simulink model "MSBR_Plant"  (R2021b)
settings: Solver=ode45  StartTime=0.0  StopTime=sim_time  MaxStep=ts_max  RelTol=1e-4
values from neighbouring files (symbols this model uses):
  a_1 = 8.7292e-2/wilson_ratio    (= 0.0087292)    [Whole_Plant_Cool_Pump_Accident_script.m]    (also in Whole_Plant_Fert_Pump_Accident_script.m; Whole_Plant_Fuel_Pump_Accident.m; Whole_Plant_Fuel_Pump_Accident_script.m; Whole_Plant_Reactivity_Accident.m)
  a_2 = 7.3787e-4/wilson_ratio    (= 7.3787e-05)    [Whole_Plant_Cool_Pump_Accident_script.m]    (also in Whole_Plant_Fert_Pump_Accident_script.m; Whole_Plant_Fuel_Pump_Accident.m; Whole_Plant_Fuel_Pump_Accident_script.m; Whole_Plant_Reactivity_Accident.m)
  a_b = 1.656e-5    (= 1.656e-05)    [Whole_Plant_Cool_Pump_Accident_script.m]    (also in Whole_Plant_Fert_Pump_Accident_script.m; Whole_Plant_Fuel_Pump_Accident.m; Whole_Plant_Fuel_Pump_Accident_script.m; Whole_Plant_Reactivity_Accident.m)
  a_f = -8.172e-5    (= -8.172e-05)    [Whole_Plant_Cool_Pump_Accident_script.m]    (also in Whole_Plant_Fert_Pump_Accident_script.m; Whole_Plant_Fuel_Pump_Accident.m; Whole_Plant_Fuel_Pump_Accident_script.m; Whole_Plant_Reactivity_Accident.m)
  a_g = 2.016e-5    (= 2.016e-05)    [Whole_Plant_Cool_Pump_Accident_script.m]    (also in Whole_Plant_Fert_Pump_Accident_script.m; Whole_Plant_Fuel_Pump_Accident.m; Whole_Plant_Fuel_Pump_Accident_script.m; Whole_Plant_Reactivity_Accident.m)
  A_s = pi()*((D_OTSG_i^2)/4) - A_w_OTSG - A_p_OTSG    [Whole_Plant_Cool_Pump_Accident_script.m]    (also in Whole_Plant_Fert_Pump_Accident_script.m; Whole_Plant_Fuel_Pump_Accident.m; Whole_Plant_Fuel_Pump_Accident_script.m; Whole_Plant_Reactivity_Accident.m)
  alpha_co = 316.2    [Whole_Plant_Cool_Pump_Accident_script.m]    (also in Whole_Plant_Fert_Pump_Accident_script.m; Whole_Plant_Fuel_Pump_Accident.m; Whole_Plant_Fuel_Pump_Accident_script.m; Whole_Plant_Reactivity_Accident.m)
  beta = [2.290e-04, 8.320e-04, 7.100e-04, 8.520e-04, 1.710e-04, 1.020e-04]    [Whole_Plant_Cool_Pump_Accident_script.m]    (also in Whole_Plant_Fert_Pump_Accident_script.m; Whole_Plant_Fuel_Pump_Accident.m; Whole_Plant_Fuel_Pump_Accident_script.m; Whole_Plant_Reactivity_Accident.m)
  beta_co = 68.0958    [Whole_Plant_Cool_Pump_Accident_script.m]    (also in Whole_Plant_Fert_Pump_Accident_script.m; Whole_Plant_Fuel_Pump_Accident.m; Whole_Plant_Fuel_Pump_Accident_script.m; Whole_Plant_Reactivity_Accident.m)
  beta_t = sum(beta)    [Whole_Plant_Cool_Pump_Accident_script.m]    (also in Whole_Plant_Fert_Pump_Accident_script.m; Whole_Plant_Fuel_Pump_Accident.m; Whole_Plant_Fuel_Pump_Accident_script.m; Whole_Plant_Reactivity_Accident.m)
  C_nc_X_A_nc = 12.8    [Whole_Plant_Cool_Pump_Accident_script.m]    (also in Whole_Plant_Fert_Pump_Accident_script.m; Whole_Plant_Fuel_Pump_Accident.m; Whole_Plant_Fuel_Pump_Accident_script.m; Whole_Plant_Reactivity_Accident.m)
  C_pcw = 0.0042    [Whole_Plant_Cool_Pump_Accident_script.m]    (also in Whole_Plant_Fert_Pump_Accident_script.m; Whole_Plant_Fuel_Pump_Accident.m; Whole_Plant_Fuel_Pump_Accident_script.m; Whole_Plant_Reactivity_Accident.m)
  C_rh_X_A_rh = 33    [Whole_Plant_Cool_Pump_Accident_script.m]    (also in Whole_Plant_Fert_Pump_Accident_script.m; Whole_Plant_Fuel_Pump_Accident.m; Whole_Plant_Fuel_Pump_Accident_script.m; Whole_Plant_Reactivity_Accident.m)
  C_v = 0.84    [Whole_Plant_Cool_Pump_Accident_script.m]    (also in Whole_Plant_Fert_Pump_Accident_script.m; Whole_Plant_Fuel_Pump_Accident.m; Whole_Plant_Fuel_Pump_Accident_script.m; Whole_Plant_Reactivity_Accident.m)
  ce1 = 1.2471e-07    [Whole_Plant_Cool_Pump_Accident_script.m]    (also in Whole_Plant_Fert_Pump_Accident_script.m; Whole_Plant_Fuel_Pump_Accident.m; Whole_Plant_Fuel_Pump_Accident_script.m; Whole_Plant_Reactivity_Accident.m)
  ce2 = 5.3816e-14    [Whole_Plant_Cool_Pump_Accident_script.m]    (also in Whole_Plant_Fert_Pump_Accident_script.m; Whole_Plant_Fuel_Pump_Accident.m; Whole_Plant_Fuel_Pump_Accident_script.m; Whole_Plant_Reactivity_Accident.m)
  ce3 = 3.3721e-08    [Whole_Plant_Cool_Pump_Accident_script.m]    (also in Whole_Plant_Fert_Pump_Accident_script.m; Whole_Plant_Fuel_Pump_Accident.m; Whole_Plant_Fuel_Pump_Accident_script.m; Whole_Plant_Reactivity_Accident.m)
  Cp_fw = XSteam('Cp_pT',P_set*10,T_fw)/1000    [Whole_Plant_Cool_Pump_Accident_script.m]    (also in Whole_Plant_Fert_Pump_Accident_script.m; Whole_Plant_Fuel_Pump_Accident.m; Whole_Plant_Fuel_Pump_Accident_script.m; Whole_Plant_Reactivity_Accident.m)
  Cp_p = Cp_sec    (= 0.001716588)    [Whole_Plant_Cool_Pump_Accident_script.m]    (also in Whole_Plant_Fert_Pump_Accident_script.m; Whole_Plant_Fuel_Pump_Accident.m; Whole_Plant_Fuel_Pump_Accident_script.m; Whole_Plant_Reactivity_Accident.m)
  Cp_rh = 0.0021520    (= 0.002152)    [Whole_Plant_Cool_Pump_Accident_script.m]    (also in Whole_Plant_Fert_Pump_Accident_script.m; Whole_Plant_Fuel_Pump_Accident.m; Whole_Plant_Fuel_Pump_Accident_script.m; Whole_Plant_Reactivity_Accident.m)
  Cp_s = XSteam('Cp_pT',P_s*10,T_s)/1000    [Whole_Plant_Cool_Pump_Accident_script.m]    (also in Whole_Plant_Fert_Pump_Accident_script.m; Whole_Plant_Fuel_Pump_Accident.m; Whole_Plant_Fuel_Pump_Accident_script.m; Whole_Plant_Reactivity_Accident.m)
  Cp_sc = XSteam('Cp_pT',P_set*10,T_sc2)/1000    [Whole_Plant_Cool_Pump_Accident_script.m]    (also in Whole_Plant_Fert_Pump_Accident_script.m; Whole_Plant_Fuel_Pump_Accident.m; Whole_Plant_Fuel_Pump_Accident_script.m; Whole_Plant_Reactivity_Accident.m)
  Cp_w = 468.992e-6    (= 0.000468992)    [Whole_Plant_Cool_Pump_Accident_script.m]    (also in Whole_Plant_Fert_Pump_Accident_script.m; Whole_Plant_Fuel_Pump_Accident.m; Whole_Plant_Fuel_Pump_Accident_script.m; Whole_Plant_Reactivity_Accident.m)
  D_it = D_ot-2*T_th    (= 0.014147)    [Whole_Plant_Cool_Pump_Accident_script.m]    (also in Whole_Plant_Fert_Pump_Accident_script.m; Whole_Plant_Fuel_Pump_Accident.m; Whole_Plant_Fuel_Pump_Accident_script.m; Whole_Plant_Reactivity_Accident.m)
  D_ot = 0.015875    [Whole_Plant_Cool_Pump_Accident_script.m]    (also in Whole_Plant_Fert_Pump_Accident_script.m; Whole_Plant_Fuel_Pump_Accident.m; Whole_Plant_Fuel_Pump_Accident_script.m; Whole_Plant_Reactivity_Accident.m)
  dHs_dPs = c(1)    [Whole_Plant_Cool_Pump_Accident_script.m]    (also in Whole_Plant_Fert_Pump_Accident_script.m; Whole_Plant_Fuel_Pump_Accident.m; Whole_Plant_Fuel_Pump_Accident_script.m; Whole_Plant_Reactivity_Accident.m)
  eta_hp_isen = 0.861    [Whole_Plant_Cool_Pump_Accident_script.m]    (also in Whole_Plant_Fert_Pump_Accident_script.m; Whole_Plant_Fuel_Pump_Accident.m; Whole_Plant_Fuel_Pump_Accident_script.m; Whole_Plant_Reactivity_Accident.m)
  eta_lp_isen = 0.861    [Whole_Plant_Cool_Pump_Accident_script.m]    (also in Whole_Plant_Fert_Pump_Accident_script.m; Whole_Plant_Fuel_Pump_Accident.m; Whole_Plant_Fuel_Pump_Accident_script.m; Whole_Plant_Reactivity_Accident.m)
  gamma_I = 5.1135e-2    (= 0.051135)    [Whole_Plant_Cool_Pump_Accident_script.m]    (also in Whole_Plant_Fert_Pump_Accident_script.m; Whole_Plant_Fuel_Pump_Accident.m; Whole_Plant_Fuel_Pump_Accident_script.m; Whole_Plant_Reactivity_Accident.m)
  gamma_Xe = 1.1628e-2    (= 0.011628)    [Whole_Plant_Cool_Pump_Accident_script.m]    (also in Whole_Plant_Fert_Pump_Accident_script.m; Whole_Plant_Fuel_Pump_Accident.m; Whole_Plant_Fuel_Pump_Accident_script.m; Whole_Plant_Reactivity_Accident.m)
  H_co0 = 0.149    [Whole_Plant_Cool_Pump_Accident_script.m]    (also in Whole_Plant_Fert_Pump_Accident_script.m; Whole_Plant_Fuel_Pump_Accident.m; Whole_Plant_Fuel_Pump_Accident_script.m; Whole_Plant_Reactivity_Accident.m)
  H_f_co0 = 0.149    [Whole_Plant_Cool_Pump_Accident_script.m]    (also in Whole_Plant_Fert_Pump_Accident_script.m; Whole_Plant_Fuel_Pump_Accident.m; Whole_Plant_Fuel_Pump_Accident_script.m; Whole_Plant_Reactivity_Accident.m)
  H_fg_co0 = 2.35    [Whole_Plant_Cool_Pump_Accident_script.m]    (also in Whole_Plant_Fert_Pump_Accident_script.m; Whole_Plant_Fuel_Pump_Accident.m; Whole_Plant_Fuel_Pump_Accident_script.m; Whole_Plant_Reactivity_Accident.m)
  H_fgrh0 = (XSteam('hV_p', P_s*1e1) - XSteam('hL_p', P_s*1e1))/1e3    [Whole_Plant_Cool_Pump_Accident_script.m]    (also in Whole_Plant_Fert_Pump_Accident_script.m; Whole_Plant_Fuel_Pump_Accident.m; Whole_Plant_Fuel_Pump_Accident_script.m; Whole_Plant_Reactivity_Accident.m)
  H_frh0 = XSteam('hL_p', P_s*1e1)/1e3    [Whole_Plant_Cool_Pump_Accident_script.m]    (also in Whole_Plant_Fert_Pump_Accident_script.m; Whole_Plant_Fuel_Pump_Accident.m; Whole_Plant_Fuel_Pump_Accident_script.m; Whole_Plant_Reactivity_Accident.m)
  h_fwh1 = 0.5927    [Whole_Plant_Cool_Pump_Accident_script.m]    (also in Whole_Plant_Fert_Pump_Accident_script.m; Whole_Plant_Fuel_Pump_Accident.m; Whole_Plant_Fuel_Pump_Accident_script.m; Whole_Plant_Reactivity_Accident.m)
  H_fwh10 = 0.46009    [Whole_Plant_Cool_Pump_Accident_script.m]    (also in Whole_Plant_Fert_Pump_Accident_script.m; Whole_Plant_Fuel_Pump_Accident.m; Whole_Plant_Fuel_Pump_Accident_script.m; Whole_Plant_Reactivity_Accident.m)
  h_fwh2 = 1.230803    [Whole_Plant_Cool_Pump_Accident_script.m]    (also in Whole_Plant_Fert_Pump_Accident_script.m; Whole_Plant_Fuel_Pump_Accident.m; Whole_Plant_Fuel_Pump_Accident_script.m; Whole_Plant_Reactivity_Accident.m)
  H_fwh20 = 0.6784    [Whole_Plant_Cool_Pump_Accident_script.m]    (also in Whole_Plant_Fert_Pump_Accident_script.m; Whole_Plant_Fuel_Pump_Accident.m; Whole_Plant_Fuel_Pump_Accident_script.m; Whole_Plant_Reactivity_Accident.m)
  H_grh0 = 2.8029    [Whole_Plant_Cool_Pump_Accident_script.m]    (also in Whole_Plant_Fert_Pump_Accident_script.m; Whole_Plant_Fuel_Pump_Accident.m; Whole_Plant_Fuel_Pump_Accident_script.m; Whole_Plant_Reactivity_Accident.m)
  H_hp_isen0 = 2.5111    [Whole_Plant_Cool_Pump_Accident_script.m]    (also in Whole_Plant_Fert_Pump_Accident_script.m; Whole_Plant_Fuel_Pump_Accident.m; Whole_Plant_Fuel_Pump_Accident_script.m; Whole_Plant_Reactivity_Accident.m)
  H_hpt_out = 2.6201    [Whole_Plant_Cool_Pump_Accident_script.m]    (also in Whole_Plant_Fert_Pump_Accident_script.m; Whole_Plant_Fuel_Pump_Accident.m; Whole_Plant_Fuel_Pump_Accident_script.m; Whole_Plant_Reactivity_Accident.m)
  H_lp_isen = 958.4*1054.35e-6/0.45359237    (= 2.22774699671)    [Whole_Plant_Cool_Pump_Accident_script.m]    (also in Whole_Plant_Fert_Pump_Accident_script.m; Whole_Plant_Fuel_Pump_Accident.m; Whole_Plant_Fuel_Pump_Accident_script.m; Whole_Plant_Reactivity_Accident.m)
  H_lpt_out = 2.3089    [Whole_Plant_Cool_Pump_Accident_script.m]    (also in Whole_Plant_Fert_Pump_Accident_script.m; Whole_Plant_Fuel_Pump_Accident.m; Whole_Plant_Fuel_Pump_Accident_script.m; Whole_Plant_Reactivity_Accident.m)
  H_nc = XSteam('h_pT', P_s*10, T_s)/1000    [Whole_Plant_Cool_Pump_Accident_script.m]    (also in Whole_Plant_Fert_Pump_Accident_script.m; Whole_Plant_Fuel_Pump_Accident.m; Whole_Plant_Fuel_Pump_Accident_script.m; Whole_Plant_Reactivity_Accident.m)
  h_pw = h_s    (= 0.02555)    [Whole_Plant_Cool_Pump_Accident_script.m]    (also in Whole_Plant_Fert_Pump_Accident_script.m; Whole_Plant_Fuel_Pump_Accident.m; Whole_Plant_Fuel_Pump_Accident_script.m; Whole_Plant_Reactivity_Accident.m)
  H_rh = 2.8115    [Whole_Plant_Cool_Pump_Accident_script.m]    (also in Whole_Plant_Fert_Pump_Accident_script.m; Whole_Plant_Fuel_Pump_Accident.m; Whole_Plant_Fuel_Pump_Accident_script.m; Whole_Plant_Reactivity_Accident.m)
  h_wb = 13349.334646671E-6    (= 0.0133493346467)    [Whole_Plant_Cool_Pump_Accident_script.m]    (also in Whole_Plant_Fert_Pump_Accident_script.m; Whole_Plant_Fuel_Pump_Accident.m; Whole_Plant_Fuel_Pump_Accident_script.m; Whole_Plant_Reactivity_Accident.m)
  h_ws = 5732.378387768E-6    (= 0.00573237838777)    [Whole_Plant_Cool_Pump_Accident_script.m]    (also in Whole_Plant_Fert_Pump_Accident_script.m; Whole_Plant_Fuel_Pump_Accident.m; Whole_Plant_Fuel_Pump_Accident_script.m; Whole_Plant_Reactivity_Accident.m)
  h_wsc = 8385.005556375E-6    (= 0.00838500555638)    [Whole_Plant_Cool_Pump_Accident_script.m]    (also in Whole_Plant_Fert_Pump_Accident_script.m; Whole_Plant_Fuel_Pump_Accident.m; Whole_Plant_Fuel_Pump_Accident_script.m; Whole_Plant_Reactivity_Accident.m)
  hA_bg = A_fert*h_bg    (= 2.76411813627)    [Whole_Plant_Cool_Pump_Accident_script.m]    (also in Whole_Plant_Fert_Pump_Accident_script.m; Whole_Plant_Fuel_Pump_Accident.m; Whole_Plant_Fuel_Pump_Accident_script.m; Whole_Plant_Reactivity_Accident.m)
  hA_co0 = 140    [Whole_Plant_Cool_Pump_Accident_script.m]    (also in Whole_Plant_Fert_Pump_Accident_script.m; Whole_Plant_Fuel_Pump_Accident.m; Whole_Plant_Fuel_Pump_Accident_script.m; Whole_Plant_Reactivity_Accident.m)
  hA_fg_dn = h_fg*A_fuel_down    [Whole_Plant_Cool_Pump_Accident_script.m]    (also in Whole_Plant_Fert_Pump_Accident_script.m; Whole_Plant_Fuel_Pump_Accident.m; Whole_Plant_Fuel_Pump_Accident_script.m; Whole_Plant_Reactivity_Accident.m)
  hA_fg_up = h_fg*A_fuel_up    [Whole_Plant_Cool_Pump_Accident_script.m]    (also in Whole_Plant_Fert_Pump_Accident_script.m; Whole_Plant_Fuel_Pump_Accident.m; Whole_Plant_Fuel_Pump_Accident_script.m; Whole_Plant_Reactivity_Accident.m)
  hA_p_bhx1 = [h_pb*A_pbhx/2,h_pb*A_pbhx/2]    [Whole_Plant_Cool_Pump_Accident_script.m]    (also in Whole_Plant_Fert_Pump_Accident_script.m; Whole_Plant_Fuel_Pump_Accident.m; Whole_Plant_Fuel_Pump_Accident_script.m; Whole_Plant_Reactivity_Accident.m)
  hA_p_bhx2 = hA_p_bhx1    [Whole_Plant_Cool_Pump_Accident_script.m]    (also in Whole_Plant_Fert_Pump_Accident_script.m; Whole_Plant_Fuel_Pump_Accident.m; Whole_Plant_Fuel_Pump_Accident_script.m; Whole_Plant_Reactivity_Accident.m)
  hA_p_bhx3 = hA_p_bhx1    [Whole_Plant_Cool_Pump_Accident_script.m]    (also in Whole_Plant_Fert_Pump_Accident_script.m; Whole_Plant_Fuel_Pump_Accident.m; Whole_Plant_Fuel_Pump_Accident_script.m; Whole_Plant_Reactivity_Accident.m)
  hA_p_bhx4 = hA_p_bhx1    [Whole_Plant_Cool_Pump_Accident_script.m]    (also in Whole_Plant_Fert_Pump_Accident_script.m; Whole_Plant_Fuel_Pump_Accident.m; Whole_Plant_Fuel_Pump_Accident_script.m; Whole_Plant_Reactivity_Accident.m)
  hA_p_fhx1 = [h_p*A_pfhx_dn/2,h_p*A_pfhx_dn/2,h_p*A_pfhx_up/2,h_p*A_pfhx_up/2]    [Whole_Plant_Cool_Pump_Accident_script.m]    (also in Whole_Plant_Fert_Pump_Accident_script.m; Whole_Plant_Fuel_Pump_Accident.m; Whole_Plant_Fuel_Pump_Accident_script.m; Whole_Plant_Reactivity_Accident.m)
  hA_p_fhx2 = hA_p_fhx1    [Whole_Plant_Cool_Pump_Accident_script.m]    (also in Whole_Plant_Fert_Pump_Accident_script.m; Whole_Plant_Fuel_Pump_Accident.m; Whole_Plant_Fuel_Pump_Accident_script.m; Whole_Plant_Reactivity_Accident.m)
  hA_p_fhx3 = hA_p_fhx1    [Whole_Plant_Cool_Pump_Accident_script.m]    (also in Whole_Plant_Fert_Pump_Accident_script.m; Whole_Plant_Fuel_Pump_Accident.m; Whole_Plant_Fuel_Pump_Accident_script.m; Whole_Plant_Reactivity_Accident.m)
  hA_p_fhx4 = hA_p_fhx1    [Whole_Plant_Cool_Pump_Accident_script.m]    (also in Whole_Plant_Fert_Pump_Accident_script.m; Whole_Plant_Fuel_Pump_Accident.m; Whole_Plant_Fuel_Pump_Accident_script.m; Whole_Plant_Reactivity_Accident.m)
  hA_s_bhx1 = [h_sb*A_sbhx/2,h_sb*A_sbhx/2]    [Whole_Plant_Cool_Pump_Accident_script.m]    (also in Whole_Plant_Fert_Pump_Accident_script.m; Whole_Plant_Fuel_Pump_Accident.m; Whole_Plant_Fuel_Pump_Accident_script.m; Whole_Plant_Reactivity_Accident.m)
  hA_s_bhx2 = hA_s_bhx1    [Whole_Plant_Cool_Pump_Accident_script.m]    (also in Whole_Plant_Fert_Pump_Accident_script.m; Whole_Plant_Fuel_Pump_Accident.m; Whole_Plant_Fuel_Pump_Accident_script.m; Whole_Plant_Reactivity_Accident.m)
  hA_s_bhx3 = hA_s_bhx1    [Whole_Plant_Cool_Pump_Accident_script.m]    (also in Whole_Plant_Fert_Pump_Accident_script.m; Whole_Plant_Fuel_Pump_Accident.m; Whole_Plant_Fuel_Pump_Accident_script.m; Whole_Plant_Reactivity_Accident.m)
  hA_s_bhx4 = hA_s_bhx1    [Whole_Plant_Cool_Pump_Accident_script.m]    (also in Whole_Plant_Fert_Pump_Accident_script.m; Whole_Plant_Fuel_Pump_Accident.m; Whole_Plant_Fuel_Pump_Accident_script.m; Whole_Plant_Reactivity_Accident.m)
  hA_s_fhx1 = [h_s*A_sfhx_up/2,h_s*A_sfhx_up/2,h_s*A_sfhx_dn/2,h_s*A_sfhx_dn/2]    [Whole_Plant_Cool_Pump_Accident_script.m]    (also in Whole_Plant_Fert_Pump_Accident_script.m; Whole_Plant_Fuel_Pump_Accident.m; Whole_Plant_Fuel_Pump_Accident_script.m; Whole_Plant_Reactivity_Accident.m)
  hA_s_fhx2 = hA_s_fhx1    [Whole_Plant_Cool_Pump_Accident_script.m]    (also in Whole_Plant_Fert_Pump_Accident_script.m; Whole_Plant_Fuel_Pump_Accident.m; Whole_Plant_Fuel_Pump_Accident_script.m; Whole_Plant_Reactivity_Accident.m)
  hA_s_fhx3 = hA_s_fhx1    [Whole_Plant_Cool_Pump_Accident_script.m]    (also in Whole_Plant_Fert_Pump_Accident_script.m; Whole_Plant_Fuel_Pump_Accident.m; Whole_Plant_Fuel_Pump_Accident_script.m; Whole_Plant_Reactivity_Accident.m)
  hA_s_fhx4 = hA_s_fhx1    [Whole_Plant_Cool_Pump_Accident_script.m]    (also in Whole_Plant_Fert_Pump_Accident_script.m; Whole_Plant_Fuel_Pump_Accident.m; Whole_Plant_Fuel_Pump_Accident_script.m; Whole_Plant_Reactivity_Accident.m)
  I_0 = gamma_I*Sigma_f_msbr*phi_0/lam_I    (= 1.30000734126e+17)    [Whole_Plant_Cool_Pump_Accident_script.m]    (also in Whole_Plant_Fert_Pump_Accident_script.m; Whole_Plant_Fuel_Pump_Accident.m; Whole_Plant_Fuel_Pump_Accident_script.m; Whole_Plant_Reactivity_Accident.m)
  k_1 = 0.5    [Whole_Plant_Cool_Pump_Accident_script.m]    (also in Whole_Plant_Fert_Pump_Accident_script.m; Whole_Plant_Fuel_Pump_Accident.m; Whole_Plant_Fuel_Pump_Accident_script.m; Whole_Plant_Reactivity_Accident.m)
  K_1 = e(1)    [Whole_Plant_Cool_Pump_Accident_script.m]    (also in Whole_Plant_Fert_Pump_Accident_script.m; Whole_Plant_Fuel_Pump_Accident.m; Whole_Plant_Fuel_Pump_Accident_script.m; Whole_Plant_Reactivity_Accident.m)
  k_1b = 0.5    [Whole_Plant_Cool_Pump_Accident_script.m]    (also in Whole_Plant_Fert_Pump_Accident_script.m; Whole_Plant_Fuel_Pump_Accident.m; Whole_Plant_Fuel_Pump_Accident_script.m; Whole_Plant_Reactivity_Accident.m)
  k_2 = 0.5    [Whole_Plant_Cool_Pump_Accident_script.m]    (also in Whole_Plant_Fert_Pump_Accident_script.m; Whole_Plant_Fuel_Pump_Accident.m; Whole_Plant_Fuel_Pump_Accident_script.m; Whole_Plant_Reactivity_Accident.m)
  k_2b = 0.5    [Whole_Plant_Cool_Pump_Accident_script.m]    (also in Whole_Plant_Fert_Pump_Accident_script.m; Whole_Plant_Fuel_Pump_Accident.m; Whole_Plant_Fuel_Pump_Accident_script.m; Whole_Plant_Reactivity_Accident.m)
  k_3 = 0.5    [Whole_Plant_Cool_Pump_Accident_script.m]    (also in Whole_Plant_Fert_Pump_Accident_script.m; Whole_Plant_Fuel_Pump_Accident.m; Whole_Plant_Fuel_Pump_Accident_script.m; Whole_Plant_Reactivity_Accident.m)
  k_4 = 0.5    [Whole_Plant_Cool_Pump_Accident_script.m]    (also in Whole_Plant_Fert_Pump_Accident_script.m; Whole_Plant_Fuel_Pump_Accident.m; Whole_Plant_Fuel_Pump_Accident_script.m; Whole_Plant_Reactivity_Accident.m)
  K_4 = b(1)    [Whole_Plant_Cool_Pump_Accident_script.m]    (also in Whole_Plant_Fert_Pump_Accident_script.m; Whole_Plant_Fuel_Pump_Accident.m; Whole_Plant_Fuel_Pump_Accident_script.m; Whole_Plant_Reactivity_Accident.m)
  K_5 = a(1)    [Whole_Plant_Cool_Pump_Accident_script.m]    (also in Whole_Plant_Fert_Pump_Accident_script.m; Whole_Plant_Fuel_Pump_Accident.m; Whole_Plant_Fuel_Pump_Accident_script.m; Whole_Plant_Reactivity_Accident.m)
  K_b = d(1)    [Whole_Plant_Cool_Pump_Accident_script.m]    (also in Whole_Plant_Fert_Pump_Accident_script.m; Whole_Plant_Fuel_Pump_Accident.m; Whole_Plant_Fuel_Pump_Accident_script.m; Whole_Plant_Reactivity_Accident.m)
  k_b1 = (K_B/2)/K    (= 0.0089463103122)    [Whole_Plant_Cool_Pump_Accident_script.m]    (also in Whole_Plant_Fert_Pump_Accident_script.m; Whole_Plant_Fuel_Pump_Accident.m; Whole_Plant_Fuel_Pump_Accident_script.m; Whole_Plant_Reactivity_Accident.m)
  k_b2 = k_b1    (= 0.0089463103122)    [Whole_Plant_Cool_Pump_Accident_script.m]    (also in Whole_Plant_Fert_Pump_Accident_script.m; Whole_Plant_Fuel_Pump_Accident.m; Whole_Plant_Fuel_Pump_Accident_script.m; Whole_Plant_Reactivity_Accident.m)
  K_bhp = 0.1634    [Whole_Plant_Cool_Pump_Accident_script.m]    (also in Whole_Plant_Fert_Pump_Accident_script.m; Whole_Plant_Fuel_Pump_Accident.m; Whole_Plant_Fuel_Pump_Accident_script.m; Whole_Plant_Reactivity_Accident.m)
  K_blp = 0.2174    [Whole_Plant_Cool_Pump_Accident_script.m]    (also in Whole_Plant_Fert_Pump_Accident_script.m; Whole_Plant_Fuel_Pump_Accident.m; Whole_Plant_Fuel_Pump_Accident_script.m; Whole_Plant_Reactivity_Accident.m)
  k_f1 = ((1 - K_G - K_B - K_Ba)/4)/K    (= 0.226055463576)    [Whole_Plant_Cool_Pump_Accident_script.m]    (also in Whole_Plant_Fert_Pump_Accident_script.m; Whole_Plant_Fuel_Pump_Accident.m; Whole_Plant_Fuel_Pump_Accident_script.m; Whole_Plant_Reactivity_Accident.m)
  k_f2 = k_f1    (= 0.226055463576)    [Whole_Plant_Cool_Pump_Accident_script.m]    (also in Whole_Plant_Fert_Pump_Accident_script.m; Whole_Plant_Fuel_Pump_Accident.m; Whole_Plant_Fuel_Pump_Accident_script.m; Whole_Plant_Reactivity_Accident.m)
  k_f3 = k_f1    (= 0.226055463576)    [Whole_Plant_Cool_Pump_Accident_script.m]    (also in Whole_Plant_Fert_Pump_Accident_script.m; Whole_Plant_Fuel_Pump_Accident.m; Whole_Plant_Fuel_Pump_Accident_script.m; Whole_Plant_Reactivity_Accident.m)
  k_f4 = k_f1    (= 0.226055463576)    [Whole_Plant_Cool_Pump_Accident_script.m]    (also in Whole_Plant_Fert_Pump_Accident_script.m; Whole_Plant_Fuel_Pump_Accident.m; Whole_Plant_Fuel_Pump_Accident_script.m; Whole_Plant_Reactivity_Accident.m)
  k_g1 = ((K_G*K_fuel)/2)/K    (= 0.0346590586566)    [Whole_Plant_Cool_Pump_Accident_script.m]    (also in Whole_Plant_Fert_Pump_Accident_script.m; Whole_Plant_Fuel_Pump_Accident.m; Whole_Plant_Fuel_Pump_Accident_script.m; Whole_Plant_Reactivity_Accident.m)
  k_g2 = k_g1    (= 0.0346590586566)    [Whole_Plant_Cool_Pump_Accident_script.m]    (also in Whole_Plant_Fert_Pump_Accident_script.m; Whole_Plant_Fuel_Pump_Accident.m; Whole_Plant_Fuel_Pump_Accident_script.m; Whole_Plant_Reactivity_Accident.m)
  k_g3 = (K_G*(1-K_fuel))/K    (= 0.00856740775781)    [Whole_Plant_Cool_Pump_Accident_script.m]    (also in Whole_Plant_Fert_Pump_Accident_script.m; Whole_Plant_Fuel_Pump_Accident.m; Whole_Plant_Fuel_Pump_Accident_script.m; Whole_Plant_Reactivity_Accident.m)
  K_sc = f(1)    [Whole_Plant_Cool_Pump_Accident_script.m]    (also in Whole_Plant_Fert_Pump_Accident_script.m; Whole_Plant_Fuel_Pump_Accident.m; Whole_Plant_Fuel_Pump_Accident_script.m; Whole_Plant_Reactivity_Accident.m)
  L = 22.0    (= 22)    [Whole_Plant_Cool_Pump_Accident_script.m]    (also in Whole_Plant_Fert_Pump_Accident_script.m; Whole_Plant_Fuel_Pump_Accident.m; Whole_Plant_Fuel_Pump_Accident_script.m; Whole_Plant_Reactivity_Accident.m)
  L_b = 1.9    [Whole_Plant_Cool_Pump_Accident_script.m]    (also in Whole_Plant_Fert_Pump_Accident_script.m; Whole_Plant_Fuel_Pump_Accident.m; Whole_Plant_Fuel_Pump_Accident_script.m; Whole_Plant_Reactivity_Accident.m)
  L_s = 16.53    [Whole_Plant_Cool_Pump_Accident_script.m]    (also in Whole_Plant_Fert_Pump_Accident_script.m; Whole_Plant_Fuel_Pump_Accident.m; Whole_Plant_Fuel_Pump_Accident_script.m; Whole_Plant_Reactivity_Accident.m)
  L_sc = L-L_b-L_s    (= 3.57)    [Whole_Plant_Cool_Pump_Accident_script.m]    (also in Whole_Plant_Fert_Pump_Accident_script.m; Whole_Plant_Fuel_Pump_Accident.m; Whole_Plant_Fuel_Pump_Accident_script.m; Whole_Plant_Reactivity_Accident.m)
  Lam = 3.3e-4    (= 0.00033)    [Whole_Plant_Cool_Pump_Accident_script.m]    (also in Whole_Plant_Fert_Pump_Accident_script.m; Whole_Plant_Fuel_Pump_Accident.m; Whole_Plant_Fuel_Pump_Accident_script.m; Whole_Plant_Reactivity_Accident.m)
  lam = [1.260e-02, 3.370e-02, 1.390e-01, 3.250e-01, 1.130e+00, 2.500e+00]    [Whole_Plant_Cool_Pump_Accident_script.m]    (also in Whole_Plant_Fert_Pump_Accident_script.m; Whole_Plant_Fuel_Pump_Accident.m; Whole_Plant_Fuel_Pump_Accident_script.m; Whole_Plant_Reactivity_Accident.m)
  lam_bubl = 2.0e-2    (= 0.02)    [Whole_Plant_Cool_Pump_Accident_script.m]    (also in Whole_Plant_Fert_Pump_Accident_script.m; Whole_Plant_Fuel_Pump_Accident.m; Whole_Plant_Fuel_Pump_Accident_script.m; Whole_Plant_Reactivity_Accident.m)
  lam_I = 2.875e-5    (= 2.875e-05)    [Whole_Plant_Cool_Pump_Accident_script.m]    (also in Whole_Plant_Fert_Pump_Accident_script.m; Whole_Plant_Fuel_Pump_Accident.m; Whole_Plant_Fuel_Pump_Accident_script.m; Whole_Plant_Reactivity_Accident.m)
  lam_Xe = 2.0916e-5    (= 2.0916e-05)    [Whole_Plant_Cool_Pump_Accident_script.m]    (also in Whole_Plant_Fert_Pump_Accident_script.m; Whole_Plant_Fuel_Pump_Accident.m; Whole_Plant_Fuel_Pump_Accident_script.m; Whole_Plant_Reactivity_Accident.m)
  m_bm = (W_b1+W_b2+W_b3+W_b4)*time_mixb    (= 2167.1636)    [Whole_Plant_Cool_Pump_Accident_script.m]    (also in Whole_Plant_Fert_Pump_Accident_script.m; Whole_Plant_Fuel_Pump_Accident.m; Whole_Plant_Fuel_Pump_Accident_script.m; Whole_Plant_Reactivity_Accident.m)
  M_cw = 65000    [Whole_Plant_Cool_Pump_Accident_script.m]    (also in Whole_Plant_Fert_Pump_Accident_script.m; Whole_Plant_Fuel_Pump_Accident.m; Whole_Plant_Fuel_Pump_Accident_script.m; Whole_Plant_Reactivity_Accident.m)
  m_fm = (W_f1+W_f2+W_f3+W_f4)*time_mixf    (= 5443.108)    [Whole_Plant_Cool_Pump_Accident_script.m]    (also in Whole_Plant_Fert_Pump_Accident_script.m; Whole_Plant_Fuel_Pump_Accident.m; Whole_Plant_Fuel_Pump_Accident_script.m; Whole_Plant_Reactivity_Accident.m)
  M_hw0 = 10000    [Whole_Plant_Cool_Pump_Accident_script.m]    (also in Whole_Plant_Fert_Pump_Accident_script.m; Whole_Plant_Fuel_Pump_Accident.m; Whole_Plant_Fuel_Pump_Accident_script.m; Whole_Plant_Reactivity_Accident.m)
  m_sm = (W_s1+W_s2+W_s3+W_s4)*time_mixs    (= 8467.056)    [Whole_Plant_Cool_Pump_Accident_script.m]    (also in Whole_Plant_Fert_Pump_Accident_script.m; Whole_Plant_Fuel_Pump_Accident.m; Whole_Plant_Fuel_Pump_Accident_script.m; Whole_Plant_Reactivity_Accident.m)
  M_stm = 0.018    [Whole_Plant_Cool_Pump_Accident_script.m]    (also in Whole_Plant_Fert_Pump_Accident_script.m; Whole_Plant_Fuel_Pump_Accident.m; Whole_Plant_Fuel_Pump_Accident_script.m; Whole_Plant_Reactivity_Accident.m)
  mcp_b1 = mass_bn*Cp_b    (= 4.17494922705)    [Whole_Plant_Cool_Pump_Accident_script.m]    (also in Whole_Plant_Fert_Pump_Accident_script.m; Whole_Plant_Fuel_Pump_Accident.m; Whole_Plant_Fuel_Pump_Accident_script.m; Whole_Plant_Reactivity_Accident.m)
  mcp_b2 = mcp_b1    (= 4.17494922705)    [Whole_Plant_Cool_Pump_Accident_script.m]    (also in Whole_Plant_Fert_Pump_Accident_script.m; Whole_Plant_Fuel_Pump_Accident.m; Whole_Plant_Fuel_Pump_Accident_script.m; Whole_Plant_Reactivity_Accident.m)
  mcp_f1 = mass_fn*Cp_f    (= 5.5019469141)    [Whole_Plant_Cool_Pump_Accident_script.m]    (also in Whole_Plant_Fert_Pump_Accident_script.m; Whole_Plant_Fuel_Pump_Accident.m; Whole_Plant_Fuel_Pump_Accident_script.m; Whole_Plant_Reactivity_Accident.m)
  mcp_f2 = mass_fn*Cp_f    (= 5.5019469141)    [Whole_Plant_Cool_Pump_Accident_script.m]    (also in Whole_Plant_Fert_Pump_Accident_script.m; Whole_Plant_Fuel_Pump_Accident.m; Whole_Plant_Fuel_Pump_Accident_script.m; Whole_Plant_Reactivity_Accident.m)
  mcp_f3 = mass_fn*Cp_f    (= 5.5019469141)    [Whole_Plant_Cool_Pump_Accident_script.m]    (also in Whole_Plant_Fert_Pump_Accident_script.m; Whole_Plant_Fuel_Pump_Accident.m; Whole_Plant_Fuel_Pump_Accident_script.m; Whole_Plant_Reactivity_Accident.m)
  mcp_f4 = mass_fn*Cp_f    (= 5.5019469141)    [Whole_Plant_Cool_Pump_Accident_script.m]    (also in Whole_Plant_Fert_Pump_Accident_script.m; Whole_Plant_Fuel_Pump_Accident.m; Whole_Plant_Fuel_Pump_Accident_script.m; Whole_Plant_Reactivity_Accident.m)
  mcp_g1 = (mass_grap*Cp_g)*K_fuel/2    (= 32.9814988203)    [Whole_Plant_Cool_Pump_Accident_script.m]    (also in Whole_Plant_Fert_Pump_Accident_script.m; Whole_Plant_Fuel_Pump_Accident.m; Whole_Plant_Fuel_Pump_Accident_script.m; Whole_Plant_Reactivity_Accident.m)
  mcp_g2 = mcp_g1    (= 32.9814988203)    [Whole_Plant_Cool_Pump_Accident_script.m]    (also in Whole_Plant_Fert_Pump_Accident_script.m; Whole_Plant_Fuel_Pump_Accident.m; Whole_Plant_Fuel_Pump_Accident_script.m; Whole_Plant_Reactivity_Accident.m)
  mcp_g3 = (mass_grap*Cp_g)*(1-K_fuel)    (= 8.15273004546)    [Whole_Plant_Cool_Pump_Accident_script.m]    (also in Whole_Plant_Fert_Pump_Accident_script.m; Whole_Plant_Fuel_Pump_Accident.m; Whole_Plant_Fuel_Pump_Accident_script.m; Whole_Plant_Reactivity_Accident.m)
  mcp_p_bhx1 = mp_bhx1*Cp_b    [Whole_Plant_Cool_Pump_Accident_script.m]    (also in Whole_Plant_Fert_Pump_Accident_script.m; Whole_Plant_Fuel_Pump_Accident.m; Whole_Plant_Fuel_Pump_Accident_script.m; Whole_Plant_Reactivity_Accident.m)
  mcp_p_bhx2 = mp_bhx2*Cp_b    [Whole_Plant_Cool_Pump_Accident_script.m]    (also in Whole_Plant_Fert_Pump_Accident_script.m; Whole_Plant_Fuel_Pump_Accident.m; Whole_Plant_Fuel_Pump_Accident_script.m; Whole_Plant_Reactivity_Accident.m)
  mcp_p_bhx3 = mp_bhx3*Cp_b    [Whole_Plant_Cool_Pump_Accident_script.m]    (also in Whole_Plant_Fert_Pump_Accident_script.m; Whole_Plant_Fuel_Pump_Accident.m; Whole_Plant_Fuel_Pump_Accident_script.m; Whole_Plant_Reactivity_Accident.m)
  ... (+213 more)
undefined symbols (not defined in the file or in its folder): C0, H_con_table, H_convap_table, H_rh_table, H_rh_table1, H_rh_table2, H_rhvap_table, H_s_table, H_table, P_con_table, P_nc_table, P_rh_table, P_rh_table1, pres_table, rho_rh_table, rho_table, SV_nc_table, SVf_nc_table, temp_table
(part 8 of 13)

== system MSBR_Plant/Nuclear Steam Supply System (NSSS)/Primary Heat Exchanger Loops (Blanket and Fuel Salt HXs)/HEAT EXCHANGER LOOP 3 ==
  Fuel HX Inlet Temperature : Inport
  Fuel Flow : Inport  Port=2
  Fuel Heat Transfer Fraction : Inport  Port=3
  Blanket HX Inlet Temperature : Inport  Port=4
  Blanket Flow : Inport  Port=5
  Blanket Heat Transfer Fraction : Inport  Port=6
  Coolant HX Inlet Temperature : Inport  Port=7
  Coolant Flow Fraction : Inport  Port=8
  Coolant hA Fraction : Inport  Port=9
  " " : Constant  Value=tau_b_fhx(3)
  Constant : Constant  Value=tau_fhx_c(3)
  Constant1 : Constant  Value=tau_fhx_fehx(3)
  Constant2 : Constant  Value=tau_fehx_b(3)
  Constant3 : Constant  Value=tau_fehx_c(3)
  Coolant OTSG-to-Fuel-HX Delay : VariableTransportDelay  MaximumDelay=1000000000000  InitialOutput=T_p6
  Coolant from Fertile HX to OTSG Delay : VariableTransportDelay  MaximumDelay=1000000000000  InitialOutput=T0_s_bhx3(2)
  Coolant from Fuel HX to Fertile HX Delay : VariableTransportDelay  MaximumDelay=100000000000  InitialOutput=T0_s_fhx3(4)
  Fertile Heat Exchanger Heat Transfer : Subsystem
  Fertile Salt from Fertile HX to Core Delay : VariableTransportDelay  MaximumDelay=1000000000000  InitialOutput=T0_p_bhx3(2)
  Fuel Heat Exchanger Heat Transfer : Subsystem
  "Fuel Salt from Fuel HX to Core Delay " : VariableTransportDelay  MaximumDelay=1000000000000  InitialOutput=T0_p_fhx3(4)
  Variable Delay for Coolant from Fertile HX to OTSG : Product  Inputs=*/
  Variable Delay for Coolant from Fuel HX to Fertile HX : Product  Inputs=*/
  Variable Delay for Coolant from OTSG to Fuel HX : Product  Inputs=*/
  Variable Delay for Fertile Salt from Fertile HX to Core : Product  Inputs=*/
  Variable Delay from Fuel HX to Core : Product  Inputs=*/
  HX3 Fuel Outlet : Outport  VectorParamsAs1DForOutWhenUnconnected=off
  HX3 Blanket Outlet : Outport  Port=2  VectorParamsAs1DForOutWhenUnconnected=off
  HX3 Coolant Outlet : Outport  Port=3  VectorParamsAs1DForOutWhenUnconnected=off
  wires:
  Fuel HX Inlet Temperature/1 -> [Tf_in]
  [Tf_in] -> Fuel Heat Exchanger Heat Transfer/1(Fuel Inlet Temp)
  Fuel Flow/1 -> [fuel_flow_frac]
  Fuel Heat Transfer Fraction/1 -> [fuel_hA_frac]
  [fuel_flow_frac] -> Fuel Heat Exchanger Heat Transfer/3(Fuel Flow Fraction)
  [fuel_hA_frac] -> Fuel Heat Exchanger Heat Transfer/4(Fuel Heat Transfer Fraction)
  [cool_flow_frac] -> Fuel Heat Exchanger Heat Transfer/5(Coolant Flow Fraction)
  [cool_hA_frac] -> Fuel Heat Exchanger Heat Transfer/6(Coolant Heat Transfer Fraction)
  [Ts_in_hx_del] -> Fuel Heat Exchanger Heat Transfer/2(Coolant Inlet Temp)
  Coolant HX Inlet Temperature/1 -> [Ts_in]
  [Ts_out_fehx_del] -> HX3 Coolant Outlet/1
  [Tp_out_phx_del] -> HX3 Fuel Outlet/1
  Blanket HX Inlet Temperature/1 -> [Tb_in]
  Blanket Flow/1 -> [blank_flow_frac]
  Blanket Heat Transfer Fraction/1 -> [blank_hA_frac]
  Fuel Heat Exchanger Heat Transfer/1(Fuel Exit Temp) -> [Tf_out]
  Fuel Heat Exchanger Heat Transfer/2(Coolant Exit Temp) -> [Ts_out_hx]
  [Ts_in_fehx_del] -> Fertile Heat Exchanger Heat Transfer/2(Coolant Inlet Temp)
  [blank_hA_frac] -> Fertile Heat Exchanger Heat Transfer/4(Blanket Heat Transfer Fraction)
  [cool_hA_frac] -> Fertile Heat Exchanger Heat Transfer/6(Coolant Heat Transfer Fraction)
  [blank_flow_frac] -> Fertile Heat Exchanger Heat Transfer/3(Blanket Flow Fraction)
  [Tb_in] -> Fertile Heat Exchanger Heat Transfer/1(Blanket Inlet Temp)
  [cool_flow_frac] -> Fertile Heat Exchanger Heat Transfer/5(Coolant Flow Fraction)
  Fertile Heat Exchanger Heat Transfer/2(Coolant Exit Temp) -> [Ts_out]
  Fertile Heat Exchanger Heat Transfer/1(Fertile Exit Temp) -> [Tb_out]
  [Tb_out_fehx_del] -> HX3 Blanket Outlet/1
  Coolant Flow Fraction/1 -> [cool_flow_frac]
  Coolant hA Fraction/1 -> [cool_hA_frac]
  Coolant OTSG-to-Fuel-HX Delay/1 -> [Ts_in_hx_del]
  Variable Delay for Coolant from Fertile HX to OTSG/1 -> Coolant from Fertile HX to OTSG Delay/2
  [Ts_out_hx] -> Coolant from Fuel HX to Fertile HX Delay/1
  Variable Delay for Coolant from Fuel HX to Fertile HX/1 -> Coolant from Fuel HX to Fertile HX Delay/2
  "Fuel Salt from Fuel HX to Core Delay "/1 -> [Tp_out_phx_del]
  [Ts_in] -> Coolant OTSG-to-Fuel-HX Delay/1
  Variable Delay for Coolant from OTSG to Fuel HX/1 -> Coolant OTSG-to-Fuel-HX Delay/2
  Variable Delay from Fuel HX to Core/1 -> "Fuel Salt from Fuel HX to Core Delay "/2
  [cool_flow_frac] -> Variable Delay for Coolant from Fuel HX to Fertile HX/2
  Fertile Salt from Fertile HX to Core Delay/1 -> [Tb_out_fehx_del]
  [Ts_out] -> Coolant from Fertile HX to OTSG Delay/1
  [cool_flow_frac] -> Variable Delay for Coolant from Fertile HX to OTSG/2
  [fuel_flow_frac] -> Variable Delay from Fuel HX to Core/2
  [blank_flow_frac] -> Variable Delay for Fertile Salt from Fertile HX to Core/2
  Coolant from Fertile HX to OTSG Delay/1 -> [Ts_out_fehx_del]
  Constant1/1 -> Variable Delay for Coolant from Fuel HX to Fertile HX/1
  " "/1 -> Variable Delay for Coolant from OTSG to Fuel HX/1
  Constant3/1 -> Variable Delay for Fertile Salt from Fertile HX to Core/1
  Variable Delay for Fertile Salt from Fertile HX to Core/1 -> Fertile Salt from Fertile HX to Core Delay/2
  [cool_flow_frac] -> Variable Delay for Coolant from OTSG to Fuel HX/2
  Constant2/1 -> Variable Delay for Coolant from Fertile HX to OTSG/1
  Constant/1 -> Variable Delay from Fuel HX to Core/1
  [Tf_out] -> "Fuel Salt from Fuel HX to Core Delay "/1
  [Tb_out] -> Fertile Salt from Fertile HX to Core Delay/1
  Coolant from Fuel HX to Fertile HX Delay/1 -> [Ts_in_fehx_del]

== system MSBR_Plant/Nuclear Steam Supply System (NSSS)/Primary Heat Exchanger Loops (Blanket and Fuel Salt HXs)/HEAT EXCHANGER LOOP 4 ==
  Fuel HX Inlet Temperature : Inport
  Fuel Flow : Inport  Port=2
  Fuel Heat Transfer Fraction : Inport  Port=3
  Blanket HX Inlet Temperature : Inport  Port=4
  Blanket Flow : Inport  Port=5
  Blanket Heat Transfer Fraction : Inport  Port=6
  Coolant HX Inlet Temperature : Inport  Port=7
  Coolant Flow Fraction : Inport  Port=8
  Coolant hA Fraction : Inport  Port=9
  " " : Constant  Value=tau_b_fhx(4)
  Constant : Constant  Value=tau_fhx_c(4)
  Constant1 : Constant  Value=tau_fhx_fehx(4)
  Constant2 : Constant  Value=tau_fehx_b(4)
  Constant3 : Constant  Value=tau_fehx_c(4)
  Coolant OTSG-to-Fuel-HX Delay : VariableTransportDelay  MaximumDelay=1000000000000  InitialOutput=T_p6
  Coolant from Fertile HX to OTSG Delay : VariableTransportDelay  MaximumDelay=1000000000000  InitialOutput=T0_s_bhx4(2)
  Coolant from Fuel HX to Fertile HX Delay : VariableTransportDelay  MaximumDelay=100000000000  InitialOutput=T0_s_fhx4(4)
  Fertile Heat Exchanger Heat Transfer : Subsystem
  Fertile Salt from Fertile HX to Core Delay : VariableTransportDelay  MaximumDelay=1000000000000  InitialOutput=T0_p_bhx4(2)
  Fuel Heat Exchanger Heat Transfer : Subsystem
  "Fuel Salt from Fuel HX to Core Delay " : VariableTransportDelay  MaximumDelay=1000000000000  InitialOutput=T0_p_fhx4(4)
  Variable Delay for Coolant from Fertile HX to OTSG : Product  Inputs=*/
  Variable Delay for Coolant from Fuel HX to Fertile HX : Product  Inputs=*/
  Variable Delay for Coolant from OTSG to Fuel HX : Product  Inputs=*/
  Variable Delay for Fertile Salt from Fertile HX to Core : Product  Inputs=*/
  Variable Delay from Fuel HX to Core : Product  Inputs=*/
  HX4 Fuel Outlet : Outport  VectorParamsAs1DForOutWhenUnconnected=off
  HX4 Blanket Outlet : Outport  Port=2  VectorParamsAs1DForOutWhenUnconnected=off
  HX4 Coolant Outlet : Outport  Port=3  VectorParamsAs1DForOutWhenUnconnected=off
  wires:
  Fuel HX Inlet Temperature/1 -> [Tf_in]
  [Tf_in] -> Fuel Heat Exchanger Heat Transfer/1(Fuel Inlet Temp)
  Fuel Flow/1 -> [fuel_flow_frac]
  Fuel Heat Transfer Fraction/1 -> [fuel_hA_frac]
  [fuel_flow_frac] -> Fuel Heat Exchanger Heat Transfer/3(Fuel Flow Fraction)
  [fuel_hA_frac] -> Fuel Heat Exchanger Heat Transfer/4(Fuel Heat Transfer Fraction)
  [cool_flow_frac] -> Fuel Heat Exchanger Heat Transfer/5(Coolant Flow Fraction)
  [cool_hA_frac] -> Fuel Heat Exchanger Heat Transfer/6(Coolant Heat Transfer Fraction)
  [Ts_in_hx_del] -> Fuel Heat Exchanger Heat Transfer/2(Coolant Inlet Temp)
  Coolant HX Inlet Temperature/1 -> [Ts_in]
  [Ts_out_fehx_del] -> HX4 Coolant Outlet/1
  [Tp_out_phx_del] -> HX4 Fuel Outlet/1
  Blanket HX Inlet Temperature/1 -> [Tb_in]
  Blanket Flow/1 -> [blank_flow_frac]
  Blanket Heat Transfer Fraction/1 -> [blank_hA_frac]
  Fuel Heat Exchanger Heat Transfer/1(Fuel Exit Temp) -> [Tf_out]
  Fuel Heat Exchanger Heat Transfer/2(Coolant Exit Temp) -> [Ts_out_hx]
  [Ts_in_fehx_del] -> Fertile Heat Exchanger Heat Transfer/2(Coolant Inlet Temp)
  [blank_hA_frac] -> Fertile Heat Exchanger Heat Transfer/4(Blanket Heat Transfer Fraction)
  [cool_hA_frac] -> Fertile Heat Exchanger Heat Transfer/6(Coolant Heat Transfer Fraction)
  [blank_flow_frac] -> Fertile Heat Exchanger Heat Transfer/3(Blanket Flow Fraction)
  [Tb_in] -> Fertile Heat Exchanger Heat Transfer/1(Blanket Inlet Temp)
  [cool_flow_frac] -> Fertile Heat Exchanger Heat Transfer/5(Coolant Flow Fraction)
  Fertile Heat Exchanger Heat Transfer/2(Coolant Exit Temp) -> [Ts_out]
  Fertile Heat Exchanger Heat Transfer/1(Fertile Exit Temp) -> [Tb_out]
  [Tb_out_fehx_del] -> HX4 Blanket Outlet/1
  Coolant hA Fraction/1 -> [cool_hA_frac]
  Coolant Flow Fraction/1 -> [cool_flow_frac]
  Variable Delay for Coolant from Fuel HX to Fertile HX/1 -> Coolant from Fuel HX to Fertile HX Delay/2
  [Ts_out_hx] -> Coolant from Fuel HX to Fertile HX Delay/1
  Variable Delay for Coolant from Fertile HX to OTSG/1 -> Coolant from Fertile HX to OTSG Delay/2
  [Tb_out] -> Fertile Salt from Fertile HX to Core Delay/1
  [Tf_out] -> "Fuel Salt from Fuel HX to Core Delay "/1
  Constant2/1 -> Variable Delay for Coolant from Fertile HX to OTSG/1
  Coolant from Fertile HX to OTSG Delay/1 -> [Ts_out_fehx_del]
  [cool_flow_frac] -> Variable Delay for Coolant from OTSG to Fuel HX/2
  Coolant from Fuel HX to Fertile HX Delay/1 -> [Ts_in_fehx_del]
  Constant1/1 -> Variable Delay for Coolant from Fuel HX to Fertile HX/1
  Constant3/1 -> Variable Delay for Fertile Salt from Fertile HX to Core/1
  [blank_flow_frac] -> Variable Delay for Fertile Salt from Fertile HX to Core/2
  Variable Delay for Fertile Salt from Fertile HX to Core/1 -> Fertile Salt from Fertile HX to Core Delay/2
  " "/1 -> Variable Delay for Coolant from OTSG to Fuel HX/1
  Constant/1 -> Variable Delay from Fuel HX to Core/1
  [fuel_flow_frac] -> Variable Delay from Fuel HX to Core/2
  [cool_flow_frac] -> Variable Delay for Coolant from Fertile HX to OTSG/2
  [Ts_out] -> Coolant from Fertile HX to OTSG Delay/1
  [cool_flow_frac] -> Variable Delay for Coolant from Fuel HX to Fertile HX/2
  Fertile Salt from Fertile HX to Core Delay/1 -> [Tb_out_fehx_del]
  Variable Delay for Coolant from OTSG to Fuel HX/1 -> Coolant OTSG-to-Fuel-HX Delay/2
  [Ts_in] -> Coolant OTSG-to-Fuel-HX Delay/1
  "Fuel Salt from Fuel HX to Core Delay "/1 -> [Tp_out_phx_del]
  Coolant OTSG-to-Fuel-HX Delay/1 -> [Ts_in_hx_del]
  Variable Delay from Fuel HX to Core/1 -> "Fuel Salt from Fuel HX to Core Delay "/2

== system MSBR_Plant/Nuclear Steam Supply System (NSSS)/Primary Pumps (Blanket and Fuel Salt)/Blanket Pump 1 ==
  note: Note that it is possible to put in a step function for the pump to reduce flow rate at a specific time. It could simulate a pipe leak/break
  note: Exponentional Function that decays with time (beginning at pump trip time). Decay rate is determined by tau_p of the pump. Final fractonal value of flow through piping is the thermal conv.
  Pump Decay Rate : Inport
  Thermal Conv : Inport  Port=2
  Pump Trip Time : Inport  Port=3
  1-D Lookup Table1 : Lookup_n-D  NumberOfTableDimensions=1  BreakpointsForDimension1=xdat  Table=ydat  InternalRulePriority=Speed  RndMeth=Simplest  InputSameDT=on
  Clock1 : Clock
  Constant : Constant
  Constant1 : Constant  Value=-1
  Divide : Product  Inputs=*/
  Math Function : Math  SaturateOnIntegerOverflow=on
  Minus : Sum  Inputs=+-
  Minus1 : Sum  Inputs=+-
  Minus3 : Sum  Inputs=+-
  Product : Product
  Scope1 : Scope
  Switch1 : Switch  Criteria=u2 > Threshold
  Switch3 : Switch  Criteria=u2 > Threshold
  To Workspace : ToWorkspace  VariableName=fert_pump_1_flow_frac  SaveFormat=Timeseries  SampleTime=-1
  To Workspace1 : ToWorkspace  VariableName=fert_pump_1_hA_frac  SaveFormat=Timeseries  SampleTime=-1
  Blanket Flow Fraction : Outport  VectorParamsAs1DForOutWhenUnconnected=off
  Blanket Heat Transfer Fraction : Outport  Port=2  VectorParamsAs1DForOutWhenUnconnected=off
  wires:
  Minus3/1 -> Switch3/2
  Product/1 -> Math Function/1
  Minus1/1 -> Product/1
  Divide/1 -> Product/2
  Constant1/1 -> Divide/1
  Constant/1 -> Switch1/1
  Clock1/1 -> Minus1/1, Minus/2
  Math Function/1 -> Switch1/3
  Switch1/1 -> Minus3/1, Switch3/1
  Minus/1 -> Switch1/2
  Pump Decay Rate/1 -> Divide/2
  Switch3/1 -> 1-D Lookup Table1/1, Scope1/1, To Workspace/1, Blanket Flow Fraction/1
  Thermal Conv/1 -> Switch3/3, Minus3/2
  Pump Trip Time/1 -> Minus1/2, Minus/1
  1-D Lookup Table1/1 -> To Workspace1/1, Blanket Heat Transfer Fraction/1

== system MSBR_Plant/Nuclear Steam Supply System (NSSS)/Primary Pumps (Blanket and Fuel Salt)/Blanket Pump 2 ==
  note: Exponentional Function that decays with time (beginning at pump trip time). Decay rate is determined by tau_p of the pump. Final fractonal value of flow through piping is the thermal conv.
  note: Note that it is possible to put in a step function for the pump to reduce flow rate at a specific time. It could simulate a pipe leak/break
  Pump Decay Rate : Inport
  Thermal Conv : Inport  Port=2
  Pump Trip Time : Inport  Port=3
  1-D Lookup Table1 : Lookup_n-D  NumberOfTableDimensions=1  BreakpointsForDimension1=xdat  Table=ydat  InternalRulePriority=Speed  RndMeth=Simplest  InputSameDT=on
  Clock1 : Clock
  Constant : Constant
  Constant1 : Constant  Value=-1
  Divide : Product  Inputs=*/
  Math Function : Math  SaturateOnIntegerOverflow=on
  Minus : Sum  Inputs=+-
  Minus1 : Sum  Inputs=+-
  Minus3 : Sum  Inputs=+-
  Product : Product
  Scope1 : Scope
  Switch1 : Switch  Criteria=u2 > Threshold
  Switch3 : Switch  Criteria=u2 > Threshold
  To Workspace : ToWorkspace  VariableName=fert_pump_2_flow_frac  SaveFormat=Timeseries  SampleTime=-1
  To Workspace1 : ToWorkspace  VariableName=fert_pump_2_hA_frac  SaveFormat=Timeseries  SampleTime=-1
  Blanket Flow Fraction : Outport  VectorParamsAs1DForOutWhenUnconnected=off
  Blanket Heat Transfer Fraction : Outport  Port=2  VectorParamsAs1DForOutWhenUnconnected=off
  wires:
  Pump Trip Time/1 -> Minus/1, Minus1/2
  Thermal Conv/1 -> Minus3/2, Switch3/3
  Pump Decay Rate/1 -> Divide/2
  Minus/1 -> Switch1/2
  Switch1/1 -> Switch3/1, Minus3/1
  Math Function/1 -> Switch1/3
  Clock1/1 -> Minus/2, Minus1/1
  Constant/1 -> Switch1/1
  Constant1/1 -> Divide/1
  Divide/1 -> Product/2
  Minus1/1 -> Product/1
  Product/1 -> Math Function/1
  Minus3/1 -> Switch3/2
  1-D Lookup Table1/1 -> To Workspace1/1, Blanket Heat Transfer Fraction/1
  Switch3/1 -> To Workspace/1, Blanket Flow Fraction/1, Scope1/1, 1-D Lookup Table1/1

== system MSBR_Plant/Nuclear Steam Supply System (NSSS)/Primary Pumps (Blanket and Fuel Salt)/Blanket Pump 3 ==
  note: Note that it is possible to put in a step function for the pump to reduce flow rate at a specific time. It could simulate a pipe leak/break
  note: Exponentional Function that decays with time (beginning at pump trip time). Decay rate is determined by tau_p of the pump. Final fractonal value of flow through piping is the thermal conv.
  Pump Decay Rate : Inport
  Thermal Conv : Inport  Port=2
  Pump Trip Time : Inport  Port=3
  1-D Lookup Table1 : Lookup_n-D  NumberOfTableDimensions=1  BreakpointsForDimension1=xdat  Table=ydat  InternalRulePriority=Speed  RndMeth=Simplest  InputSameDT=on
  Clock1 : Clock
  Constant : Constant
  Constant1 : Constant  Value=-1
  Divide : Product  Inputs=*/
  Math Function : Math  SaturateOnIntegerOverflow=on
  Minus : Sum  Inputs=+-
  Minus1 : Sum  Inputs=+-
  Minus3 : Sum  Inputs=+-
  Product : Product
  Scope1 : Scope
  Switch1 : Switch  Criteria=u2 > Threshold
  Switch3 : Switch  Criteria=u2 > Threshold
  To Workspace : ToWorkspace  VariableName=fert_pump_3_flow_frac  SaveFormat=Timeseries  SampleTime=-1
  To Workspace1 : ToWorkspace  VariableName=fert_pump_3_hA_frac  SaveFormat=Timeseries  SampleTime=-1
  Blanket Flow Fraction : Outport  VectorParamsAs1DForOutWhenUnconnected=off
  Blanket Heat Transfer Fraction : Outport  Port=2  VectorParamsAs1DForOutWhenUnconnected=off
  wires:
  Minus3/1 -> Switch3/2
  Product/1 -> Math Function/1
  Minus1/1 -> Product/1
  Divide/1 -> Product/2
  Constant1/1 -> Divide/1
  Constant/1 -> Switch1/1
  Clock1/1 -> Minus1/1, Minus/2
  Math Function/1 -> Switch1/3
  Switch1/1 -> Minus3/1, Switch3/1
  Minus/1 -> Switch1/2
  Pump Decay Rate/1 -> Divide/2
  Thermal Conv/1 -> Switch3/3, Minus3/2
  Pump Trip Time/1 -> Minus1/2, Minus/1
  1-D Lookup Table1/1 -> To Workspace1/1, Blanket Heat Transfer Fraction/1
  Switch3/1 -> 1-D Lookup Table1/1, Scope1/1, To Workspace/1, Blanket Flow Fraction/1

== system MSBR_Plant/Nuclear Steam Supply System (NSSS)/Primary Pumps (Blanket and Fuel Salt)/Blanket Pump 4 ==
  note: Exponentional Function that decays with time (beginning at pump trip time). Decay rate is determined by tau_p of the pump. Final fractonal value of flow through piping is the thermal conv.
  note: Note that it is possible to put in a step function for the pump to reduce flow rate at a specific time. It could simulate a pipe leak/break
  Pump Decay Rate : Inport
  Thermal Conv : Inport  Port=2
  Pump Trip Time : Inport  Port=3
  1-D Lookup Table1 : Lookup_n-D  NumberOfTableDimensions=1  BreakpointsForDimension1=xdat  Table=ydat  InternalRulePriority=Speed  RndMeth=Simplest  InputSameDT=on
  Clock1 : Clock
  Constant : Constant
  Constant1 : Constant  Value=-1
  Divide : Product  Inputs=*/
  Math Function : Math  SaturateOnIntegerOverflow=on
  Minus : Sum  Inputs=+-
  Minus1 : Sum  Inputs=+-
  Minus3 : Sum  Inputs=+-
  Product : Product
  Scope1 : Scope
  Switch1 : Switch  Criteria=u2 > Threshold
  Switch3 : Switch  Criteria=u2 > Threshold
  To Workspace : ToWorkspace  VariableName=fert_pump_4_flow_frac  SaveFormat=Timeseries  SampleTime=-1
  To Workspace1 : ToWorkspace  VariableName=fert_pump_4_hA_frac  SaveFormat=Timeseries  SampleTime=-1
  Blanket Flow Fraction : Outport  VectorParamsAs1DForOutWhenUnconnected=off
  Blanket Heat Transfer Fraction : Outport  Port=2  VectorParamsAs1DForOutWhenUnconnected=off
  wires:
  Pump Trip Time/1 -> Minus/1, Minus1/2
  Thermal Conv/1 -> Minus3/2, Switch3/3
  Pump Decay Rate/1 -> Divide/2
  Minus/1 -> Switch1/2
  Switch1/1 -> Switch3/1, Minus3/1
  Math Function/1 -> Switch1/3
  Clock1/1 -> Minus/2, Minus1/1
  Constant/1 -> Switch1/1
  Constant1/1 -> Divide/1
  Divide/1 -> Product/2
  Minus1/1 -> Product/1
  Product/1 -> Math Function/1
  Minus3/1 -> Switch3/2
  1-D Lookup Table1/1 -> To Workspace1/1, Blanket Heat Transfer Fraction/1
  Switch3/1 -> To Workspace/1, Blanket Flow Fraction/1, Scope1/1, 1-D Lookup Table1/1
